simulink model "bit32cpu"  (R2020a)
settings: Solver=VariableStepAuto  StartTime=0.0  StopTime=10.0  RelTol=1e-3
libraries: simulink_extras x392
(part 10 of 63)

== system bit32cpu/ALU/Multiplier/Subsystem2/Subsystem1/Subsystem3 ==
  In1 : Inport
  In2 : Inport  Port=2
  In3 : Inport  Port=3
  In4 : Inport  Port=4
  In5 : Inport  Port=5
  In6 : Inport  Port=6
  In7 : Inport  Port=7
  In8 : Inport  Port=8
  Logical Operator{,1..15} (16 alike) : Logic  AllPortsSameDT=off  OutDataTypeStr=boolean
  Subsystem : Subsystem
  Subsystem1 : Subsystem
  Subsystem10 : Subsystem
  Subsystem11 : Subsystem
  Subsystem12 : Subsystem
  Subsystem13 : Subsystem
  Subsystem14 : Subsystem
  Subsystem2 : Subsystem
  Subsystem3 : Subsystem
  Subsystem4 : Subsystem
  Subsystem5 : Subsystem
  Subsystem6 : Subsystem
  Subsystem7 : Subsystem
  Subsystem8 : Subsystem
  Subsystem9 : Subsystem
  Out1 : Outport
  Out2 : Outport  Port=2
  Out3 : Outport  Port=3
  Out4 : Outport  Port=4
  Out5 : Outport  Port=5
  Out6 : Outport  Port=6
  Out7 : Outport  Port=7
  Out8 : Outport  Port=8
  Out9 : Outport  Port=9
  wires:
  Logical Operator3/1 -> Out9/1
  Subsystem2/1(Out1) -> Out7/1
  Logical Operator4/1 -> Subsystem6/1(In1)
  Subsystem1/2(Out2) -> Subsystem10/1(In1)
  Subsystem9/2(Out2) -> Subsystem14/2(In2)
  Subsystem7/1(Out1) -> Out5/1
  Logical Operator11/1 -> Subsystem1/3(In3)
  Logical Operator10/1 -> Subsystem3/3(In3)
  Subsystem4/1(Out1) -> Out6/1
  In4/1 -> Logical Operator15/2, Logical Operator11/2, Logical Operator7/2, Logical Operator3/2
  Subsystem14/1(Out1) -> Out2/1
  Subsystem14/2(Out2) -> Out1/1
  Logical Operator8/1 -> Subsystem8/1(In1)
  Subsystem3/2(Out2) -> Subsystem5/1(In1)
  In5/1 -> Logical Operator12/1, Logical Operator13/1, Logical Operator14/1, Logical Operator15/1
  In7/1 -> Logical Operator4/1, Logical Operator5/1, Logical Operator6/1, Logical Operator7/1
  Subsystem8/2(Out2) -> Subsystem12/1(In1)
  Subsystem13/1(Out1) -> Out4/1
  Subsystem/1(Out1) -> Out8/1
  Subsystem9/1(Out1) -> Out3/1
  Subsystem11/1(Out1) -> Subsystem8/3(In3)
  Logical Operator2/1 -> Subsystem/1(In1)
  In8/1 -> Logical Operator/1, Logical Operator1/1, Logical Operator2/1, Logical Operator3/1
  Logical Operator6/1 -> Subsystem1/2(In2)
  Subsystem12/1(Out1) -> Subsystem9/3(In3)
  In2/1 -> Logical Operator9/2, Logical Operator13/2, Logical Operator5/2, Logical Operator1/2
  Subsystem5/2(Out2) -> Subsystem13/2(In2)
  Logical Operator12/1 -> Subsystem9/1(In1)
  Subsystem2/2(Out2) -> Subsystem10/2(In2)
  Logical Operator14/1 -> Subsystem6/3(In3)
  In3/1 -> Logical Operator6/2, Logical Operator14/2, Logical Operator10/2, Logical Operator2/2
  Subsystem4/2(Out2) -> Subsystem5/2(In2)
  Subsystem/2(Out2) -> Subsystem2/2(In2)
  In1/1 -> Logical Operator12/2, Logical Operator8/2, Logical Operator4/2, Logical Operator/2
  In6/1 -> Logical Operator8/1, Logical Operator9/1, Logical Operator10/1, Logical Operator11/1
  Logical Operator/1 -> Subsystem3/1(In1)
  Logical Operator9/1 -> Subsystem6/2(In2)
  Subsystem12/2(Out2) -> Subsystem14/1(In1)
  Subsystem10/2(Out2) -> Subsystem7/3(In3)
  Logical Operator13/1 -> Subsystem8/2(In2)
  Logical Operator1/1 -> Subsystem1/1(In1)
  Subsystem1/1(Out1) -> Subsystem2/1(In1)
  Subsystem6/2(Out2) -> Subsystem11/1(In1)
  Logical Operator5/1 -> Subsystem3/2(In2)
  Logical Operator7/1 -> Subsystem/2(In2)
  Subsystem11/2(Out2) -> Subsystem9/2(In2)
  Subsystem6/1(Out1) -> Subsystem7/1(In1)
  Subsystem8/1(Out1) -> Subsystem13/1(In1)
  Subsystem13/2(Out2) -> Subsystem12/2(In2)
  Subsystem5/1(Out1) -> Subsystem7/2(In2)
  Logical Operator15/1 -> Subsystem4/1(In1)
  Subsystem3/1(Out1) -> Subsystem4/2(In2)
  Subsystem7/2(Out2) -> Subsystem11/2(In2)
  Subsystem10/1(Out1) -> Subsystem4/3(In3)

== system bit32cpu/ALU/Multiplier/Subsystem2/Subsystem1/Subsystem4 ==
  In1 : Inport
  In2 : Inport  Port=2
  In3 : Inport  Port=3
  In4 : Inport  Port=4
  In5 : Inport  Port=5
  In6 : Inport  Port=6
  In7 : Inport  Port=7
  In8 : Inport  Port=8
  In9 : Inport  Port=9
  In10 : Inport  Port=10
  In11 : Inport  Port=11
  In12 : Inport  Port=12
  In13 : Inport  Port=13
  In14 : Inport  Port=14
  In15 : Inport  Port=15
  In16 : Inport  Port=16
  Constant16 : Constant  Value=0
  Subsystem : Subsystem
  Subsystem4 : Subsystem
  Out1 : Outport
  Out2 : Outport  Port=2
  Out3 : Outport  Port=3
  Out4 : Outport  Port=4
  Out5 : Outport  Port=5
  Out6 : Outport  Port=6
  Out7 : Outport  Port=7
  Out8 : Outport  Port=8
  Out9 : Outport  Port=9
  wires:
  Subsystem/3(Out3) -> Out7/1
  Subsystem4/5(Out5) -> Out5/1
  Subsystem4/3(Out3) -> Out3/1
  Subsystem4/1(Out1) -> Out1/1
  Subsystem/2(Out2) -> Out6/1
  Subsystem4/2(Out2) -> Out2/1
  Subsystem/1(Out1) -> Subsystem4/5(In5)
  Subsystem4/4(Out4) -> Out4/1
  Subsystem/5(Out5) -> Out9/1
  Constant16/1 -> Subsystem/5(In5)
  Subsystem/4(Out4) -> Out8/1
  In1/1 -> Subsystem4/1(In1)
  In2/1 -> Subsystem4/2(In2)
  In3/1 -> Subsystem4/3(In3)
  In4/1 -> Subsystem4/4(In4)
  In5/1 -> Subsystem/1(In1)
  In6/1 -> Subsystem/2(In2)
  In7/1 -> Subsystem/3(In3)
  In8/1 -> Subsystem/4(In4)
  In9/1 -> Subsystem4/6(In6)
  In10/1 -> Subsystem4/7(In7)
  In11/1 -> Subsystem4/8(In8)
  In12/1 -> Subsystem4/9(In9)
  In13/1 -> Subsystem/6(In6)
  In14/1 -> Subsystem/7(In7)
  In15/1 -> Subsystem/8(In8)
  In16/1 -> Subsystem/9(In9)

== system bit32cpu/ALU/Multiplier/Subsystem2/Subsystem1/Subsystem5 ==
  In1 : Inport
  In2 : Inport  Port=2
  In3 : Inport  Port=3
  In4 : Inport  Port=4
  In5 : Inport  Port=5
  In6 : Inport  Port=6
  In7 : Inport  Port=7
  In8 : Inport  Port=8
  In9 : Inport  Port=9
  In10 : Inport  Port=10
  In11 : Inport  Port=11
  In12 : Inport  Port=12
  In13 : Inport  Port=13
  In14 : Inport  Port=14
  In15 : Inport  Port=15
  In16 : Inport  Port=16
  Constant16 : Constant  Value=0
  Subsystem : Subsystem
  Subsystem4 : Subsystem
  Out1 : Outport
  Out2 : Outport  Port=2
  Out3 : Outport  Port=3
  Out4 : Outport  Port=4
  Out5 : Outport  Port=5
  Out6 : Outport  Port=6
  Out7 : Outport  Port=7
  Out8 : Outport  Port=8
  Out9 : Outport  Port=9
  wires:
  Subsystem/3(Out3) -> Out7/1
  Subsystem4/5(Out5) -> Out5/1
  Subsystem4/3(Out3) -> Out3/1
  Subsystem4/1(Out1) -> Out1/1
  Subsystem/2(Out2) -> Out6/1
  Subsystem4/2(Out2) -> Out2/1
  Subsystem/1(Out1) -> Subsystem4/5(In5)
  Subsystem4/4(Out4) -> Out4/1
  Subsystem/5(Out5) -> Out9/1
  Constant16/1 -> Subsystem/5(In5)
  Subsystem/4(Out4) -> Out8/1
  In1/1 -> Subsystem4/1(In1)
  In2/1 -> Subsystem4/2(In2)
  In3/1 -> Subsystem4/3(In3)
  In4/1 -> Subsystem4/4(In4)
  In5/1 -> Subsystem/1(In1)
  In6/1 -> Subsystem/2(In2)
  In7/1 -> Subsystem/3(In3)
  In8/1 -> Subsystem/4(In4)
  In9/1 -> Subsystem4/6(In6)
  In10/1 -> Subsystem4/7(In7)
  In11/1 -> Subsystem4/8(In8)
  In12/1 -> Subsystem4/9(In9)
  In13/1 -> Subsystem/6(In6)
  In14/1 -> Subsystem/7(In7)
  In15/1 -> Subsystem/8(In8)
  In16/1 -> Subsystem/9(In9)

== system bit32cpu/ALU/Multiplier/Subsystem2/Subsystem1/Subsystem6 ==
  In1 : Inport
  In2 : Inport  Port=2
  In3 : Inport  Port=3
  In4 : Inport  Port=4
  In5 : Inport  Port=5
  In6 : Inport  Port=6
  In7 : Inport  Port=7
  In8 : Inport  Port=8
  In9 : Inport  Port=9
  In10 : Inport  Port=10
  In11 : Inport  Port=11
  In12 : Inport  Port=12
  In13 : Inport  Port=13
  In14 : Inport  Port=14
  In15 : Inport  Port=15
  In16 : Inport  Port=16
  Constant : Constant  Value=0
  Subsystem : Subsystem
  Subsystem4 : Subsystem
  Out1 : Outport
  Out2 : Outport  Port=2
  Out3 : Outport  Port=3
  Out4 : Outport  Port=4
  Out5 : Outport  Port=5
  Out6 : Outport  Port=6
  Out7 : Outport  Port=7
  Out8 : Outport  Port=8
  Out9 : Outport  Port=9
  wires:
  Subsystem/3(Out3) -> Out7/1
  Subsystem4/5(Out5) -> Out5/1
  Subsystem4/3(Out3) -> Out3/1
  Subsystem4/1(Out1) -> Out1/1
  Subsystem/2(Out2) -> Out6/1
  Subsystem4/2(Out2) -> Out2/1
  Subsystem/1(Out1) -> Subsystem4/5(In5)
  Subsystem4/4(Out4) -> Out4/1
  Subsystem/5(Out5) -> Out9/1
  Constant/1 -> Subsystem/5(In5)
  Subsystem/4(Out4) -> Out8/1
  In1/1 -> Subsystem4/1(In1)
  In2/1 -> Subsystem4/2(In2)
  In3/1 -> Subsystem4/3(In3)
  In4/1 -> Subsystem4/4(In4)
  In5/1 -> Subsystem/1(In1)
  In6/1 -> Subsystem/2(In2)
  In7/1 -> Subsystem/3(In3)
  In8/1 -> Subsystem/4(In4)
  In9/1 -> Subsystem4/6(In6)
  In10/1 -> Subsystem4/7(In7)
  In11/1 -> Subsystem4/8(In8)
  In12/1 -> Subsystem4/9(In9)
  In13/1 -> Subsystem/6(In6)
  In14/1 -> Subsystem/7(In7)
  In15/1 -> Subsystem/8(In8)
  In16/1 -> Subsystem/9(In9)

== system bit32cpu/ALU/Multiplier/Subsystem2/Subsystem2/Subsystem1 ==
  In1 : Inport
  In2 : Inport  Port=2
  In3 : Inport  Port=3
  In4 : Inport  Port=4
  In5 : Inport  Port=5
  In6 : Inport  Port=6
  In7 : Inport  Port=7
  In8 : Inport  Port=8
  Logical Operator{,1..15} (16 alike) : Logic  AllPortsSameDT=off  OutDataTypeStr=boolean
  Subsystem : Subsystem
  Subsystem1 : Subsystem
  Subsystem10 : Subsystem
  Subsystem11 : Subsystem
  Subsystem12 : Subsystem
  Subsystem13 : Subsystem
  Subsystem14 : Subsystem
  Subsystem2 : Subsystem
  Subsystem3 : Subsystem
  Subsystem4 : Subsystem
  Subsystem5 : Subsystem
  Subsystem6 : Subsystem
  Subsystem7 : Subsystem
  Subsystem8 : Subsystem
  Subsystem9 : Subsystem
  Out1 : Outport
  Out2 : Outport  Port=2
  Out3 : Outport  Port=3
  Out4 : Outport  Port=4
  Out5 : Outport  Port=5
  Out6 : Outport  Port=6
  Out7 : Outport  Port=7
  Out8 : Outport  Port=8
  Out9 : Outport  Port=9
  wires:
  Logical Operator3/1 -> Out9/1
  Subsystem2/1(Out1) -> Out7/1
  Logical Operator4/1 -> Subsystem6/1(In1)
  Subsystem1/2(Out2) -> Subsystem10/1(In1)
  Subsystem9/2(Out2) -> Subsystem14/2(In2)
  Subsystem7/1(Out1) -> Out5/1
  Logical Operator11/1 -> Subsystem1/3(In3)
  Logical Operator10/1 -> Subsystem3/3(In3)
  Subsystem4/1(Out1) -> Out6/1
  In4/1 -> Logical Operator15/2, Logical Operator11/2, Logical Operator7/2, Logical Operator3/2
  Subsystem14/1(Out1) -> Out2/1
  Subsystem14/2(Out2) -> Out1/1
  Logical Operator8/1 -> Subsystem8/1(In1)
  Subsystem3/2(Out2) -> Subsystem5/1(In1)
  In5/1 -> Logical Operator12/1, Logical Operator13/1, Logical Operator14/1, Logical Operator15/1
  In7/1 -> Logical Operator4/1, Logical Operator5/1, Logical Operator6/1, Logical Operator7/1
  Subsystem8/2(Out2) -> Subsystem12/1(In1)
  Subsystem13/1(Out1) -> Out4/1
  Subsystem/1(Out1) -> Out8/1
  Subsystem9/1(Out1) -> Out3/1
  Subsystem11/1(Out1) -> Subsystem8/3(In3)
  Logical Operator2/1 -> Subsystem/1(In1)
  In8/1 -> Logical Operator/1, Logical Operator1/1, Logical Operator2/1, Logical Operator3/1
  Logical Operator6/1 -> Subsystem1/2(In2)
  Subsystem12/1(Out1) -> Subsystem9/3(In3)
  In2/1 -> Logical Operator9/2, Logical Operator13/2, Logical Operator5/2, Logical Operator1/2
  Subsystem5/2(Out2) -> Subsystem13/2(In2)
  Logical Operator12/1 -> Subsystem9/1(In1)
  Subsystem2/2(Out2) -> Subsystem10/2(In2)
  Logical Operator14/1 -> Subsystem6/3(In3)
  In3/1 -> Logical Operator6/2, Logical Operator14/2, Logical Operator10/2, Logical Operator2/2
  Subsystem4/2(Out2) -> Subsystem5/2(In2)
  Subsystem/2(Out2) -> Subsystem2/2(In2)
  In1/1 -> Logical Operator12/2, Logical Operator8/2, Logical Operator4/2, Logical Operator/2
  In6/1 -> Logical Operator8/1, Logical Operator9/1, Logical Operator10/1, Logical Operator11/1
  Logical Operator/1 -> Subsystem3/1(In1)
  Logical Operator9/1 -> Subsystem6/2(In2)
  Subsystem12/2(Out2) -> Subsystem14/1(In1)
  Subsystem10/2(Out2) -> Subsystem7/3(In3)
  Logical Operator13/1 -> Subsystem8/2(In2)
  Logical Operator1/1 -> Subsystem1/1(In1)
  Subsystem1/1(Out1) -> Subsystem2/1(In1)
  Subsystem6/2(Out2) -> Subsystem11/1(In1)
  Logical Operator5/1 -> Subsystem3/2(In2)
  Logical Operator7/1 -> Subsystem/2(In2)
  Subsystem11/2(Out2) -> Subsystem9/2(In2)
  Subsystem6/1(Out1) -> Subsystem7/1(In1)
  Subsystem8/1(Out1) -> Subsystem13/1(In1)
  Subsystem13/2(Out2) -> Subsystem12/2(In2)
  Subsystem5/1(Out1) -> Subsystem7/2(In2)
  Logical Operator15/1 -> Subsystem4/1(In1)
  Subsystem3/1(Out1) -> Subsystem4/2(In2)
  Subsystem7/2(Out2) -> Subsystem11/2(In2)
  Subsystem10/1(Out1) -> Subsystem4/3(In3)

== system bit32cpu/ALU/Multiplier/Subsystem2/Subsystem2/Subsystem15 ==
  In1 : Inport
  In2 : Inport  Port=2
  In3 : Inport  Port=3
  In4 : Inport  Port=4
  In5 : Inport  Port=5
  In6 : Inport  Port=6
  In7 : Inport  Port=7
  In8 : Inport  Port=8
  Logical Operator{,1..15} (16 alike) : Logic  AllPortsSameDT=off  OutDataTypeStr=boolean
  Subsystem : Subsystem
  Subsystem1 : Subsystem
  Subsystem10 : Subsystem
  Subsystem11 : Subsystem
  Subsystem12 : Subsystem
  Subsystem13 : Subsystem
  Subsystem14 : Subsystem
  Subsystem2 : Subsystem
  Subsystem3 : Subsystem
  Subsystem4 : Subsystem
  Subsystem5 : Subsystem
  Subsystem6 : Subsystem
  Subsystem7 : Subsystem
  Subsystem8 : Subsystem
  Subsystem9 : Subsystem
  Out1 : Outport
  Out2 : Outport  Port=2
  Out3 : Outport  Port=3
  Out4 : Outport  Port=4
  Out5 : Outport  Port=5
  Out6 : Outport  Port=6
  Out7 : Outport  Port=7
  Out8 : Outport  Port=8
  Out9 : Outport  Port=9
  wires:
  Logical Operator3/1 -> Out9/1
  Subsystem2/1(Out1) -> Out7/1
  Logical Operator4/1 -> Subsystem6/1(In1)
  Subsystem1/2(Out2) -> Subsystem10/1(In1)
  Subsystem9/2(Out2) -> Subsystem14/2(In2)
  Subsystem7/1(Out1) -> Out5/1
  Logical Operator11/1 -> Subsystem1/3(In3)
  Logical Operator10/1 -> Subsystem3/3(In3)
  Subsystem4/1(Out1) -> Out6/1
  In4/1 -> Logical Operator15/2, Logical Operator11/2, Logical Operator7/2, Logical Operator3/2
  Subsystem14/1(Out1) -> Out2/1
  Subsystem14/2(Out2) -> Out1/1
  Logical Operator8/1 -> Subsystem8/1(In1)
  Subsystem3/2(Out2) -> Subsystem5/1(In1)
  In5/1 -> Logical Operator12/1, Logical Operator13/1, Logical Operator14/1, Logical Operator15/1
  In7/1 -> Logical Operator4/1, Logical Operator5/1, Logical Operator6/1, Logical Operator7/1
  Subsystem8/2(Out2) -> Subsystem12/1(In1)
  Subsystem13/1(Out1) -> Out4/1
  Subsystem/1(Out1) -> Out8/1
  Subsystem9/1(Out1) -> Out3/1
  Subsystem11/1(Out1) -> Subsystem8/3(In3)
  Logical Operator2/1 -> Subsystem/1(In1)
  In8/1 -> Logical Operator/1, Logical Operator1/1, Logical Operator2/1, Logical Operator3/1
  Logical Operator6/1 -> Subsystem1/2(In2)
  Subsystem12/1(Out1) -> Subsystem9/3(In3)
  In2/1 -> Logical Operator9/2, Logical Operator13/2, Logical Operator5/2, Logical Operator1/2
  Subsystem5/2(Out2) -> Subsystem13/2(In2)
  Logical Operator12/1 -> Subsystem9/1(In1)
  Subsystem2/2(Out2) -> Subsystem10/2(In2)
  Logical Operator14/1 -> Subsystem6/3(In3)
  In3/1 -> Logical Operator6/2, Logical Operator14/2, Logical Operator10/2, Logical Operator2/2
  Subsystem4/2(Out2) -> Subsystem5/2(In2)
  Subsystem/2(Out2) -> Subsystem2/2(In2)
  In1/1 -> Logical Operator12/2, Logical Operator8/2, Logical Operator4/2, Logical Operator/2
  In6/1 -> Logical Operator8/1, Logical Operator9/1, Logical Operator10/1, Logical Operator11/1
  Logical Operator/1 -> Subsystem3/1(In1)
  Logical Operator9/1 -> Subsystem6/2(In2)
  Subsystem12/2(Out2) -> Subsystem14/1(In1)
  Subsystem10/2(Out2) -> Subsystem7/3(In3)
  Logical Operator13/1 -> Subsystem8/2(In2)
  Logical Operator1/1 -> Subsystem1/1(In1)
  Subsystem1/1(Out1) -> Subsystem2/1(In1)
  Subsystem6/2(Out2) -> Subsystem11/1(In1)
  Logical Operator5/1 -> Subsystem3/2(In2)
  Logical Operator7/1 -> Subsystem/2(In2)
  Subsystem11/2(Out2) -> Subsystem9/2(In2)
  Subsystem6/1(Out1) -> Subsystem7/1(In1)
  Subsystem8/1(Out1) -> Subsystem13/1(In1)
  Subsystem13/2(Out2) -> Subsystem12/2(In2)
  Subsystem5/1(Out1) -> Subsystem7/2(In2)
  Logical Operator15/1 -> Subsystem4/1(In1)
  Subsystem3/1(Out1) -> Subsystem4/2(In2)
  Subsystem7/2(Out2) -> Subsystem11/2(In2)
  Subsystem10/1(Out1) -> Subsystem4/3(In3)

== system bit32cpu/ALU/Multiplier/Subsystem2/Subsystem2/Subsystem2 ==
  In1 : Inport
  In2 : Inport  Port=2
  In3 : Inport  Port=3
  In4 : Inport  Port=4
  In5 : Inport  Port=5
  In6 : Inport  Port=6
  In7 : Inport  Port=7
  In8 : Inport  Port=8
  Logical Operator{,1..15} (16 alike) : Logic  AllPortsSameDT=off  OutDataTypeStr=boolean
  Subsystem : Subsystem
  Subsystem1 : Subsystem
  Subsystem10 : Subsystem
  Subsystem11 : Subsystem
  Subsystem12 : Subsystem
  Subsystem13 : Subsystem
  Subsystem14 : Subsystem
  Subsystem2 : Subsystem
  Subsystem3 : Subsystem
  Subsystem4 : Subsystem
  Subsystem5 : Subsystem
  Subsystem6 : Subsystem
  Subsystem7 : Subsystem
  Subsystem8 : Subsystem
  Subsystem9 : Subsystem
  Out1 : Outport
  Out2 : Outport  Port=2
  Out3 : Outport  Port=3
  Out4 : Outport  Port=4
  Out5 : Outport  Port=5
  Out6 : Outport  Port=6
  Out7 : Outport  Port=7
  Out8 : Outport  Port=8
  Out9 : Outport  Port=9
  wires:
  Logical Operator3/1 -> Out9/1
  Subsystem2/1(Out1) -> Out7/1
  Logical Operator4/1 -> Subsystem6/1(In1)
  Subsystem1/2(Out2) -> Subsystem10/1(In1)
  Subsystem9/2(Out2) -> Subsystem14/2(In2)
  Subsystem7/1(Out1) -> Out5/1
  Logical Operator11/1 -> Subsystem1/3(In3)
  Logical Operator10/1 -> Subsystem3/3(In3)
  Subsystem4/1(Out1) -> Out6/1
  In4/1 -> Logical Operator15/2, Logical Operator11/2, Logical Operator7/2, Logical Operator3/2
  Subsystem14/1(Out1) -> Out2/1
  Subsystem14/2(Out2) -> Out1/1
  Logical Operator8/1 -> Subsystem8/1(In1)
  Subsystem3/2(Out2) -> Subsystem5/1(In1)
  In5/1 -> Logical Operator12/1, Logical Operator13/1, Logical Operator14/1, Logical Operator15/1
  In7/1 -> Logical Operator4/1, Logical Operator5/1, Logical Operator6/1, Logical Operator7/1
  Subsystem8/2(Out2) -> Subsystem12/1(In1)
  Subsystem13/1(Out1) -> Out4/1
  Subsystem/1(Out1) -> Out8/1
  Subsystem9/1(Out1) -> Out3/1
  Subsystem11/1(Out1) -> Subsystem8/3(In3)
  Logical Operator2/1 -> Subsystem/1(In1)
  In8/1 -> Logical Operator/1, Logical Operator1/1, Logical Operator2/1, Logical Operator3/1
  Logical Operator6/1 -> Subsystem1/2(In2)
  Subsystem12/1(Out1) -> Subsystem9/3(In3)
  In2/1 -> Logical Operator9/2, Logical Operator13/2, Logical Operator5/2, Logical Operator1/2
  Subsystem5/2(Out2) -> Subsystem13/2(In2)
  Logical Operator12/1 -> Subsystem9/1(In1)
  Subsystem2/2(Out2) -> Subsystem10/2(In2)
  Logical Operator14/1 -> Subsystem6/3(In3)
  In3/1 -> Logical Operator6/2, Logical Operator14/2, Logical Operator10/2, Logical Operator2/2
  Subsystem4/2(Out2) -> Subsystem5/2(In2)
  Subsystem/2(Out2) -> Subsystem2/2(In2)
  In1/1 -> Logical Operator12/2, Logical Operator8/2, Logical Operator4/2, Logical Operator/2
  In6/1 -> Logical Operator8/1, Logical Operator9/1, Logical Operator10/1, Logical Operator11/1
  Logical Operator/1 -> Subsystem3/1(In1)
  Logical Operator9/1 -> Subsystem6/2(In2)
  Subsystem12/2(Out2) -> Subsystem14/1(In1)
  Subsystem10/2(Out2) -> Subsystem7/3(In3)
  Logical Operator13/1 -> Subsystem8/2(In2)
  Logical Operator1/1 -> Subsystem1/1(In1)
  Subsystem1/1(Out1) -> Subsystem2/1(In1)
  Subsystem6/2(Out2) -> Subsystem11/1(In1)
  Logical Operator5/1 -> Subsystem3/2(In2)
  Logical Operator7/1 -> Subsystem/2(In2)
  Subsystem11/2(Out2) -> Subsystem9/2(In2)
  Subsystem6/1(Out1) -> Subsystem7/1(In1)
  Subsystem8/1(Out1) -> Subsystem13/1(In1)
  Subsystem13/2(Out2) -> Subsystem12/2(In2)
  Subsystem5/1(Out1) -> Subsystem7/2(In2)
  Logical Operator15/1 -> Subsystem4/1(In1)
  Subsystem3/1(Out1) -> Subsystem4/2(In2)
  Subsystem7/2(Out2) -> Subsystem11/2(In2)
  Subsystem10/1(Out1) -> Subsystem4/3(In3)

== system bit32cpu/ALU/Multiplier/Subsystem2/Subsystem2/Subsystem3 ==
  In1 : Inport
  In2 : Inport  Port=2
  In3 : Inport  Port=3
  In4 : Inport  Port=4
  In5 : Inport  Port=5
  In6 : Inport  Port=6
  In7 : Inport  Port=7
  In8 : Inport  Port=8
  Logical Operator{,1..15} (16 alike) : Logic  AllPortsSameDT=off  OutDataTypeStr=boolean
  Subsystem : Subsystem
  Subsystem1 : Subsystem
  Subsystem10 : Subsystem
  Subsystem11 : Subsystem
  Subsystem12 : Subsystem
  Subsystem13 : Subsystem
  Subsystem14 : Subsystem
  Subsystem2 : Subsystem
  Subsystem3 : Subsystem
  Subsystem4 : Subsystem
  Subsystem5 : Subsystem
  Subsystem6 : Subsystem
  Subsystem7 : Subsystem
  Subsystem8 : Subsystem
  Subsystem9 : Subsystem
  Out1 : Outport
  Out2 : Outport  Port=2
  Out3 : Outport  Port=3
  Out4 : Outport  Port=4
  Out5 : Outport  Port=5
  Out6 : Outport  Port=6
  Out7 : Outport  Port=7
  Out8 : Outport  Port=8
  Out9 : Outport  Port=9
  wires:
  Logical Operator3/1 -> Out9/1
  Subsystem2/1(Out1) -> Out7/1
  Logical Operator4/1 -> Subsystem6/1(In1)
  Subsystem1/2(Out2) -> Subsystem10/1(In1)
  Subsystem9/2(Out2) -> Subsystem14/2(In2)
  Subsystem7/1(Out1) -> Out5/1
  Logical Operator11/1 -> Subsystem1/3(In3)
  Logical Operator10/1 -> Subsystem3/3(In3)
  Subsystem4/1(Out1) -> Out6/1
  In4/1 -> Logical Operator15/2, Logical Operator11/2, Logical Operator7/2, Logical Operator3/2
  Subsystem14/1(Out1) -> Out2/1
  Subsystem14/2(Out2) -> Out1/1
  Logical Operator8/1 -> Subsystem8/1(In1)
  Subsystem3/2(Out2) -> Subsystem5/1(In1)
  In5/1 -> Logical Operator12/1, Logical Operator13/1, Logical Operator14/1, Logical Operator15/1
  In7/1 -> Logical Operator4/1, Logical Operator5/1, Logical Operator6/1, Logical Operator7/1
  Subsystem8/2(Out2) -> Subsystem12/1(In1)
  Subsystem13/1(Out1) -> Out4/1
  Subsystem/1(Out1) -> Out8/1
  Subsystem9/1(Out1) -> Out3/1
  Subsystem11/1(Out1) -> Subsystem8/3(In3)
  Logical Operator2/1 -> Subsystem/1(In1)
  In8/1 -> Logical Operator/1, Logical Operator1/1, Logical Operator2/1, Logical Operator3/1
  Logical Operator6/1 -> Subsystem1/2(In2)
  Subsystem12/1(Out1) -> Subsystem9/3(In3)
  In2/1 -> Logical Operator9/2, Logical Operator13/2, Logical Operator5/2, Logical Operator1/2
  Subsystem5/2(Out2) -> Subsystem13/2(In2)
  Logical Operator12/1 -> Subsystem9/1(In1)
  Subsystem2/2(Out2) -> Subsystem10/2(In2)
  Logical Operator14/1 -> Subsystem6/3(In3)
  In3/1 -> Logical Operator6/2, Logical Operator14/2, Logical Operator10/2, Logical Operator2/2
  Subsystem4/2(Out2) -> Subsystem5/2(In2)
  Subsystem/2(Out2) -> Subsystem2/2(In2)
  In1/1 -> Logical Operator12/2, Logical Operator8/2, Logical Operator4/2, Logical Operator/2
  In6/1 -> Logical Operator8/1, Logical Operator9/1, Logical Operator10/1, Logical Operator11/1
  Logical Operator/1 -> Subsystem3/1(In1)
  Logical Operator9/1 -> Subsystem6/2(In2)
  Subsystem12/2(Out2) -> Subsystem14/1(In1)
  Subsystem10/2(Out2) -> Subsystem7/3(In3)
  Logical Operator13/1 -> Subsystem8/2(In2)
  Logical Operator1/1 -> Subsystem1/1(In1)
  Subsystem1/1(Out1) -> Subsystem2/1(In1)
  Subsystem6/2(Out2) -> Subsystem11/1(In1)
  Logical Operator5/1 -> Subsystem3/2(In2)
  Logical Operator7/1 -> Subsystem/2(In2)
  Subsystem11/2(Out2) -> Subsystem9/2(In2)
  Subsystem6/1(Out1) -> Subsystem7/1(In1)
  Subsystem8/1(Out1) -> Subsystem13/1(In1)
  Subsystem13/2(Out2) -> Subsystem12/2(In2)
  Subsystem5/1(Out1) -> Subsystem7/2(In2)
  Logical Operator15/1 -> Subsystem4/1(In1)
  Subsystem3/1(Out1) -> Subsystem4/2(In2)
  Subsystem7/2(Out2) -> Subsystem11/2(In2)
  Subsystem10/1(Out1) -> Subsystem4/3(In3)

== system bit32cpu/ALU/Multiplier/Subsystem2/Subsystem2/Subsystem4 ==
  In1 : Inport
  In2 : Inport  Port=2
  In3 : Inport  Port=3
  In4 : Inport  Port=4
  In5 : Inport  Port=5
  In6 : Inport  Port=6
  In7 : Inport  Port=7
  In8 : Inport  Port=8
  In9 : Inport  Port=9
  In10 : Inport  Port=10
  In11 : Inport  Port=11
  In12 : Inport  Port=12
  In13 : Inport  Port=13
  In14 : Inport  Port=14
  In15 : Inport  Port=15
  In16 : Inport  Port=16
  Constant16 : Constant  Value=0
  Subsystem : Subsystem
  Subsystem4 : Subsystem
  Out1 : Outport
  Out2 : Outport  Port=2
  Out3 : Outport  Port=3
  Out4 : Outport  Port=4
  Out5 : Outport  Port=5
  Out6 : Outport  Port=6
  Out7 : Outport  Port=7
  Out8 : Outport  Port=8
  Out9 : Outport  Port=9
  wires:
  Subsystem/3(Out3) -> Out7/1
  Subsystem4/5(Out5) -> Out5/1
  Subsystem4/3(Out3) -> Out3/1
  Subsystem4/1(Out1) -> Out1/1
  Subsystem/2(Out2) -> Out6/1
  Subsystem4/2(Out2) -> Out2/1
  Subsystem/1(Out1) -> Subsystem4/5(In5)
  Subsystem4/4(Out4) -> Out4/1
  Subsystem/5(Out5) -> Out9/1
  Constant16/1 -> Subsystem/5(In5)
  Subsystem/4(Out4) -> Out8/1
  In1/1 -> Subsystem4/1(In1)
  In2/1 -> Subsystem4/2(In2)
  In3/1 -> Subsystem4/3(In3)
  In4/1 -> Subsystem4/4(In4)
  In5/1 -> Subsystem/1(In1)
  In6/1 -> Subsystem/2(In2)
  In7/1 -> Subsystem/3(In3)
  In8/1 -> Subsystem/4(In4)
  In9/1 -> Subsystem4/6(In6)
  In10/1 -> Subsystem4/7(In7)
  In11/1 -> Subsystem4/8(In8)
  In12/1 -> Subsystem4/9(In9)
  In13/1 -> Subsystem/6(In6)
  In14/1 -> Subsystem/7(In7)
  In15/1 -> Subsystem/8(In8)
  In16/1 -> Subsystem/9(In9)

== system bit32cpu/ALU/Multiplier/Subsystem2/Subsystem2/Subsystem5 ==
  In1 : Inport
  In2 : Inport  Port=2
  In3 : Inport  Port=3
  In4 : Inport  Port=4
  In5 : Inport  Port=5
  In6 : Inport  Port=6
  In7 : Inport  Port=7
  In8 : Inport  Port=8
  In9 : Inport  Port=9
  In10 : Inport  Port=10
  In11 : Inport  Port=11
  In12 : Inport  Port=12
  In13 : Inport  Port=13
  In14 : Inport  Port=14
  In15 : Inport  Port=15
  In16 : Inport  Port=16
  Constant16 : Constant  Value=0
  Subsystem : Subsystem
  Subsystem4 : Subsystem
  Out1 : Outport
  Out2 : Outport  Port=2
  Out3 : Outport  Port=3
  Out4 : Outport  Port=4
  Out5 : Outport  Port=5
  Out6 : Outport  Port=6
  Out7 : Outport  Port=7
  Out8 : Outport  Port=8
  Out9 : Outport  Port=9
  wires:
  Subsystem/3(Out3) -> Out7/1
  Subsystem4/5(Out5) -> Out5/1
  Subsystem4/3(Out3) -> Out3/1
  Subsystem4/1(Out1) -> Out1/1
  Subsystem/2(Out2) -> Out6/1
  Subsystem4/2(Out2) -> Out2/1
  Subsystem/1(Out1) -> Subsystem4/5(In5)
  Subsystem4/4(Out4) -> Out4/1
  Subsystem/5(Out5) -> Out9/1
  Constant16/1 -> Subsystem/5(In5)
  Subsystem/4(Out4) -> Out8/1
  In1/1 -> Subsystem4/1(In1)
  In2/1 -> Subsystem4/2(In2)
  In3/1 -> Subsystem4/3(In3)
  In4/1 -> Subsystem4/4(In4)
  In5/1 -> Subsystem/1(In1)
  In6/1 -> Subsystem/2(In2)
  In7/1 -> Subsystem/3(In3)
  In8/1 -> Subsystem/4(In4)
  In9/1 -> Subsystem4/6(In6)
  In10/1 -> Subsystem4/7(In7)
  In11/1 -> Subsystem4/8(In8)
  In12/1 -> Subsystem4/9(In9)
  In13/1 -> Subsystem/6(In6)
  In14/1 -> Subsystem/7(In7)
  In15/1 -> Subsystem/8(In8)
  In16/1 -> Subsystem/9(In9)

== system bit32cpu/ALU/Multiplier/Subsystem2/Subsystem2/Subsystem6 ==
  In1 : Inport
  In2 : Inport  Port=2
  In3 : Inport  Port=3
  In4 : Inport  Port=4
  In5 : Inport  Port=5
  In6 : Inport  Port=6
  In7 : Inport  Port=7
  In8 : Inport  Port=8
  In9 : Inport  Port=9
  In10 : Inport  Port=10
  In11 : Inport  Port=11
  In12 : Inport  Port=12
  In13 : Inport  Port=13
  In14 : Inport  Port=14
  In15 : Inport  Port=15
  In16 : Inport  Port=16
  Constant : Constant  Value=0
  Subsystem : Subsystem
  Subsystem4 : Subsystem
  Out1 : Outport
  Out2 : Outport  Port=2
  Out3 : Outport  Port=3
  Out4 : Outport  Port=4
  Out5 : Outport  Port=5
  Out6 : Outport  Port=6
  Out7 : Outport  Port=7
  Out8 : Outport  Port=8
  Out9 : Outport  Port=9
  wires:
  Subsystem/3(Out3) -> Out7/1
  Subsystem4/5(Out5) -> Out5/1
  Subsystem4/3(Out3) -> Out3/1
  Subsystem4/1(Out1) -> Out1/1
  Subsystem/2(Out2) -> Out6/1
  Subsystem4/2(Out2) -> Out2/1
  Subsystem/1(Out1) -> Subsystem4/5(In5)
  Subsystem4/4(Out4) -> Out4/1
  Subsystem/5(Out5) -> Out9/1
  Constant/1 -> Subsystem/5(In5)
  Subsystem/4(Out4) -> Out8/1
  In1/1 -> Subsystem4/1(In1)
  In2/1 -> Subsystem4/2(In2)
  In3/1 -> Subsystem4/3(In3)
  In4/1 -> Subsystem4/4(In4)
  In5/1 -> Subsystem/1(In1)
  In6/1 -> Subsystem/2(In2)
  In7/1 -> Subsystem/3(In3)
  In8/1 -> Subsystem/4(In4)
  In9/1 -> Subsystem4/6(In6)
  In10/1 -> Subsystem4/7(In7)
  In11/1 -> Subsystem4/8(In8)
  In12/1 -> Subsystem4/9(In9)
  In13/1 -> Subsystem/6(In6)
  In14/1 -> Subsystem/7(In7)
  In15/1 -> Subsystem/8(In8)
  In16/1 -> Subsystem/9(In9)

== system bit32cpu/ALU/Multiplier/Subsystem2/Subsystem3/Subsystem1 ==
  In1 : Inport
  In2 : Inport  Port=2
  In3 : Inport  Port=3
  In4 : Inport  Port=4
  In5 : Inport  Port=5
  In6 : Inport  Port=6
  In7 : Inport  Port=7
  In8 : Inport  Port=8
  Logical Operator{,1..15} (16 alike) : Logic  AllPortsSameDT=off  OutDataTypeStr=boolean
  Subsystem : Subsystem
  Subsystem1 : Subsystem
  Subsystem10 : Subsystem
  Subsystem11 : Subsystem
  Subsystem12 : Subsystem
  Subsystem13 : Subsystem
  Subsystem14 : Subsystem
  Subsystem2 : Subsystem
  Subsystem3 : Subsystem
  Subsystem4 : Subsystem
  Subsystem5 : Subsystem
  Subsystem6 : Subsystem
  Subsystem7 : Subsystem
  Subsystem8 : Subsystem
  Subsystem9 : Subsystem
  Out1 : Outport
  Out2 : Outport  Port=2
  Out3 : Outport  Port=3
  Out4 : Outport  Port=4
  Out5 : Outport  Port=5
  Out6 : Outport  Port=6
  Out7 : Outport  Port=7
  Out8 : Outport  Port=8
  Out9 : Outport  Port=9
  wires:
  Logical Operator3/1 -> Out9/1
  Subsystem2/1(Out1) -> Out7/1
  Logical Operator4/1 -> Subsystem6/1(In1)
  Subsystem1/2(Out2) -> Subsystem10/1(In1)
  Subsystem9/2(Out2) -> Subsystem14/2(In2)
  Subsystem7/1(Out1) -> Out5/1
  Logical Operator11/1 -> Subsystem1/3(In3)
  Logical Operator10/1 -> Subsystem3/3(In3)
  Subsystem4/1(Out1) -> Out6/1
  In4/1 -> Logical Operator15/2, Logical Operator11/2, Logical Operator7/2, Logical Operator3/2
  Subsystem14/1(Out1) -> Out2/1
  Subsystem14/2(Out2) -> Out1/1
  Logical Operator8/1 -> Subsystem8/1(In1)
  Subsystem3/2(Out2) -> Subsystem5/1(In1)
  In5/1 -> Logical Operator12/1, Logical Operator13/1, Logical Operator14/1, Logical Operator15/1
  In7/1 -> Logical Operator4/1, Logical Operator5/1, Logical Operator6/1, Logical Operator7/1
  Subsystem8/2(Out2) -> Subsystem12/1(In1)
  Subsystem13/1(Out1) -> Out4/1
  Subsystem/1(Out1) -> Out8/1
  Subsystem9/1(Out1) -> Out3/1
  Subsystem11/1(Out1) -> Subsystem8/3(In3)
  Logical Operator2/1 -> Subsystem/1(In1)
  In8/1 -> Logical Operator/1, Logical Operator1/1, Logical Operator2/1, Logical Operator3/1
  Logical Operator6/1 -> Subsystem1/2(In2)
  Subsystem12/1(Out1) -> Subsystem9/3(In3)
  In2/1 -> Logical Operator9/2, Logical Operator13/2, Logical Operator5/2, Logical Operator1/2
  Subsystem5/2(Out2) -> Subsystem13/2(In2)
  Logical Operator12/1 -> Subsystem9/1(In1)
  Subsystem2/2(Out2) -> Subsystem10/2(In2)
  Logical Operator14/1 -> Subsystem6/3(In3)
  In3/1 -> Logical Operator6/2, Logical Operator14/2, Logical Operator10/2, Logical Operator2/2
  Subsystem4/2(Out2) -> Subsystem5/2(In2)
  Subsystem/2(Out2) -> Subsystem2/2(In2)
  In1/1 -> Logical Operator12/2, Logical Operator8/2, Logical Operator4/2, Logical Operator/2
  In6/1 -> Logical Operator8/1, Logical Operator9/1, Logical Operator10/1, Logical Operator11/1
  Logical Operator/1 -> Subsystem3/1(In1)
  Logical Operator9/1 -> Subsystem6/2(In2)
  Subsystem12/2(Out2) -> Subsystem14/1(In1)
  Subsystem10/2(Out2) -> Subsystem7/3(In3)
  Logical Operator13/1 -> Subsystem8/2(In2)
  Logical Operator1/1 -> Subsystem1/1(In1)
  Subsystem1/1(Out1) -> Subsystem2/1(In1)
  Subsystem6/2(Out2) -> Subsystem11/1(In1)
  Logical Operator5/1 -> Subsystem3/2(In2)
  Logical Operator7/1 -> Subsystem/2(In2)
  Subsystem11/2(Out2) -> Subsystem9/2(In2)
  Subsystem6/1(Out1) -> Subsystem7/1(In1)
  Subsystem8/1(Out1) -> Subsystem13/1(In1)
  Subsystem13/2(Out2) -> Subsystem12/2(In2)
  Subsystem5/1(Out1) -> Subsystem7/2(In2)
  Logical Operator15/1 -> Subsystem4/1(In1)
  Subsystem3/1(Out1) -> Subsystem4/2(In2)
  Subsystem7/2(Out2) -> Subsystem11/2(In2)
  Subsystem10/1(Out1) -> Subsystem4/3(In3)

== system bit32cpu/ALU/Multiplier/Subsystem2/Subsystem3/Subsystem15 ==
  In1 : Inport
  In2 : Inport  Port=2
  In3 : Inport  Port=3
  In4 : Inport  Port=4
  In5 : Inport  Port=5
  In6 : Inport  Port=6
  In7 : Inport  Port=7
  In8 : Inport  Port=8
  Logical Operator{,1..15} (16 alike) : Logic  AllPortsSameDT=off  OutDataTypeStr=boolean
  Subsystem : Subsystem
  Subsystem1 : Subsystem
  Subsystem10 : Subsystem
  Subsystem11 : Subsystem
  Subsystem12 : Subsystem
  Subsystem13 : Subsystem
  Subsystem14 : Subsystem
  Subsystem2 : Subsystem
  Subsystem3 : Subsystem
  Subsystem4 : Subsystem
  Subsystem5 : Subsystem
  Subsystem6 : Subsystem
  Subsystem7 : Subsystem
  Subsystem8 : Subsystem
  Subsystem9 : Subsystem
  Out1 : Outport
  Out2 : Outport  Port=2
  Out3 : Outport  Port=3
  Out4 : Outport  Port=4
  Out5 : Outport  Port=5
  Out6 : Outport  Port=6
  Out7 : Outport  Port=7
  Out8 : Outport  Port=8
  Out9 : Outport  Port=9
  wires:
  Logical Operator3/1 -> Out9/1
  Subsystem2/1(Out1) -> Out7/1
  Logical Operator4/1 -> Subsystem6/1(In1)
  Subsystem1/2(Out2) -> Subsystem10/1(In1)
  Subsystem9/2(Out2) -> Subsystem14/2(In2)
  Subsystem7/1(Out1) -> Out5/1
  Logical Operator11/1 -> Subsystem1/3(In3)
  Logical Operator10/1 -> Subsystem3/3(In3)
  Subsystem4/1(Out1) -> Out6/1
  In4/1 -> Logical Operator15/2, Logical Operator11/2, Logical Operator7/2, Logical Operator3/2
  Subsystem14/1(Out1) -> Out2/1
  Subsystem14/2(Out2) -> Out1/1
  Logical Operator8/1 -> Subsystem8/1(In1)
  Subsystem3/2(Out2) -> Subsystem5/1(In1)
  In5/1 -> Logical Operator12/1, Logical Operator13/1, Logical Operator14/1, Logical Operator15/1
  In7/1 -> Logical Operator4/1, Logical Operator5/1, Logical Operator6/1, Logical Operator7/1
  Subsystem8/2(Out2) -> Subsystem12/1(In1)
  Subsystem13/1(Out1) -> Out4/1
  Subsystem/1(Out1) -> Out8/1
  Subsystem9/1(Out1) -> Out3/1
  Subsystem11/1(Out1) -> Subsystem8/3(In3)
  Logical Operator2/1 -> Subsystem/1(In1)
  In8/1 -> Logical Operator/1, Logical Operator1/1, Logical Operator2/1, Logical Operator3/1
  Logical Operator6/1 -> Subsystem1/2(In2)
  Subsystem12/1(Out1) -> Subsystem9/3(In3)
  In2/1 -> Logical Operator9/2, Logical Operator13/2, Logical Operator5/2, Logical Operator1/2
  Subsystem5/2(Out2) -> Subsystem13/2(In2)
  Logical Operator12/1 -> Subsystem9/1(In1)
  Subsystem2/2(Out2) -> Subsystem10/2(In2)
  Logical Operator14/1 -> Subsystem6/3(In3)
  In3/1 -> Logical Operator6/2, Logical Operator14/2, Logical Operator10/2, Logical Operator2/2
  Subsystem4/2(Out2) -> Subsystem5/2(In2)
  Subsystem/2(Out2) -> Subsystem2/2(In2)
  In1/1 -> Logical Operator12/2, Logical Operator8/2, Logical Operator4/2, Logical Operator/2
  In6/1 -> Logical Operator8/1, Logical Operator9/1, Logical Operator10/1, Logical Operator11/1
  Logical Operator/1 -> Subsystem3/1(In1)
  Logical Operator9/1 -> Subsystem6/2(In2)
  Subsystem12/2(Out2) -> Subsystem14/1(In1)
  Subsystem10/2(Out2) -> Subsystem7/3(In3)
  Logical Operator13/1 -> Subsystem8/2(In2)
  Logical Operator1/1 -> Subsystem1/1(In1)
  Subsystem1/1(Out1) -> Subsystem2/1(In1)
  Subsystem6/2(Out2) -> Subsystem11/1(In1)
  Logical Operator5/1 -> Subsystem3/2(In2)
  Logical Operator7/1 -> Subsystem/2(In2)
  Subsystem11/2(Out2) -> Subsystem9/2(In2)
  Subsystem6/1(Out1) -> Subsystem7/1(In1)
  Subsystem8/1(Out1) -> Subsystem13/1(In1)
  Subsystem13/2(Out2) -> Subsystem12/2(In2)
  Subsystem5/1(Out1) -> Subsystem7/2(In2)
  Logical Operator15/1 -> Subsystem4/1(In1)
  Subsystem3/1(Out1) -> Subsystem4/2(In2)
  Subsystem7/2(Out2) -> Subsystem11/2(In2)
  Subsystem10/1(Out1) -> Subsystem4/3(In3)

== system bit32cpu/ALU/Multiplier/Subsystem2/Subsystem3/Subsystem2 ==
  In1 : Inport
  In2 : Inport  Port=2
  In3 : Inport  Port=3
  In4 : Inport  Port=4
  In5 : Inport  Port=5
  In6 : Inport  Port=6
  In7 : Inport  Port=7
  In8 : Inport  Port=8
  Logical Operator{,1..15} (16 alike) : Logic  AllPortsSameDT=off  OutDataTypeStr=boolean
  Subsystem : Subsystem
  Subsystem1 : Subsystem
  Subsystem10 : Subsystem
  Subsystem11 : Subsystem
  Subsystem12 : Subsystem
  Subsystem13 : Subsystem
  Subsystem14 : Subsystem
  Subsystem2 : Subsystem
  Subsystem3 : Subsystem
  Subsystem4 : Subsystem
  Subsystem5 : Subsystem
  Subsystem6 : Subsystem
  Subsystem7 : Subsystem
  Subsystem8 : Subsystem
  Subsystem9 : Subsystem
  Out1 : Outport
  Out2 : Outport  Port=2
  Out3 : Outport  Port=3
  Out4 : Outport  Port=4
  Out5 : Outport  Port=5
  Out6 : Outport  Port=6
  Out7 : Outport  Port=7
  Out8 : Outport  Port=8
  Out9 : Outport  Port=9
  wires:
  Logical Operator3/1 -> Out9/1
  Subsystem2/1(Out1) -> Out7/1
  Logical Operator4/1 -> Subsystem6/1(In1)
  Subsystem1/2(Out2) -> Subsystem10/1(In1)
  Subsystem9/2(Out2) -> Subsystem14/2(In2)
  Subsystem7/1(Out1) -> Out5/1
  Logical Operator11/1 -> Subsystem1/3(In3)
  Logical Operator10/1 -> Subsystem3/3(In3)
  Subsystem4/1(Out1) -> Out6/1
  In4/1 -> Logical Operator15/2, Logical Operator11/2, Logical Operator7/2, Logical Operator3/2
  Subsystem14/1(Out1) -> Out2/1
  Subsystem14/2(Out2) -> Out1/1
  Logical Operator8/1 -> Subsystem8/1(In1)
  Subsystem3/2(Out2) -> Subsystem5/1(In1)
  In5/1 -> Logical Operator12/1, Logical Operator13/1, Logical Operator14/1, Logical Operator15/1
  In7/1 -> Logical Operator4/1, Logical Operator5/1, Logical Operator6/1, Logical Operator7/1
  Subsystem8/2(Out2) -> Subsystem12/1(In1)
  Subsystem13/1(Out1) -> Out4/1
  Subsystem/1(Out1) -> Out8/1
  Subsystem9/1(Out1) -> Out3/1
  Subsystem11/1(Out1) -> Subsystem8/3(In3)
  Logical Operator2/1 -> Subsystem/1(In1)
  In8/1 -> Logical Operator/1, Logical Operator1/1, Logical Operator2/1, Logical Operator3/1
  Logical Operator6/1 -> Subsystem1/2(In2)
  Subsystem12/1(Out1) -> Subsystem9/3(In3)
  In2/1 -> Logical Operator9/2, Logical Operator13/2, Logical Operator5/2, Logical Operator1/2
  Subsystem5/2(Out2) -> Subsystem13/2(In2)
  Logical Operator12/1 -> Subsystem9/1(In1)
  Subsystem2/2(Out2) -> Subsystem10/2(In2)
  Logical Operator14/1 -> Subsystem6/3(In3)
  In3/1 -> Logical Operator6/2, Logical Operator14/2, Logical Operator10/2, Logical Operator2/2
  Subsystem4/2(Out2) -> Subsystem5/2(In2)
  Subsystem/2(Out2) -> Subsystem2/2(In2)
  In1/1 -> Logical Operator12/2, Logical Operator8/2, Logical Operator4/2, Logical Operator/2
  In6/1 -> Logical Operator8/1, Logical Operator9/1, Logical Operator10/1, Logical Operator11/1
  Logical Operator/1 -> Subsystem3/1(In1)
  Logical Operator9/1 -> Subsystem6/2(In2)
  Subsystem12/2(Out2) -> Subsystem14/1(In1)
  Subsystem10/2(Out2) -> Subsystem7/3(In3)
  Logical Operator13/1 -> Subsystem8/2(In2)
  Logical Operator1/1 -> Subsystem1/1(In1)
  Subsystem1/1(Out1) -> Subsystem2/1(In1)
  Subsystem6/2(Out2) -> Subsystem11/1(In1)
  Logical Operator5/1 -> Subsystem3/2(In2)
  Logical Operator7/1 -> Subsystem/2(In2)
  Subsystem11/2(Out2) -> Subsystem9/2(In2)
  Subsystem6/1(Out1) -> Subsystem7/1(In1)
  Subsystem8/1(Out1) -> Subsystem13/1(In1)
  Subsystem13/2(Out2) -> Subsystem12/2(In2)
  Subsystem5/1(Out1) -> Subsystem7/2(In2)
  Logical Operator15/1 -> Subsystem4/1(In1)
  Subsystem3/1(Out1) -> Subsystem4/2(In2)
  Subsystem7/2(Out2) -> Subsystem11/2(In2)
  Subsystem10/1(Out1) -> Subsystem4/3(In3)

== system bit32cpu/ALU/Multiplier/Subsystem2/Subsystem3/Subsystem3 ==
  In1 : Inport
  In2 : Inport  Port=2
  In3 : Inport  Port=3
  In4 : Inport  Port=4
  In5 : Inport  Port=5
  In6 : Inport  Port=6
  In7 : Inport  Port=7
  In8 : Inport  Port=8
  Logical Operator{,1..15} (16 alike) : Logic  AllPortsSameDT=off  OutDataTypeStr=boolean
  Subsystem : Subsystem
  Subsystem1 : Subsystem
  Subsystem10 : Subsystem
  Subsystem11 : Subsystem
  Subsystem12 : Subsystem
  Subsystem13 : Subsystem
  Subsystem14 : Subsystem
  Subsystem2 : Subsystem
  Subsystem3 : Subsystem
  Subsystem4 : Subsystem
  Subsystem5 : Subsystem
  Subsystem6 : Subsystem
  Subsystem7 : Subsystem
  Subsystem8 : Subsystem
  Subsystem9 : Subsystem
  Out1 : Outport
  Out2 : Outport  Port=2
  Out3 : Outport  Port=3
  Out4 : Outport  Port=4
  Out5 : Outport  Port=5
  Out6 : Outport  Port=6
  Out7 : Outport  Port=7
  Out8 : Outport  Port=8
  Out9 : Outport  Port=9
  wires:
  Logical Operator3/1 -> Out9/1
  Subsystem2/1(Out1) -> Out7/1
  Logical Operator4/1 -> Subsystem6/1(In1)
  Subsystem1/2(Out2) -> Subsystem10/1(In1)
  Subsystem9/2(Out2) -> Subsystem14/2(In2)
  Subsystem7/1(Out1) -> Out5/1
  Logical Operator11/1 -> Subsystem1/3(In3)
  Logical Operator10/1 -> Subsystem3/3(In3)
  Subsystem4/1(Out1) -> Out6/1
  In4/1 -> Logical Operator15/2, Logical Operator11/2, Logical Operator7/2, Logical Operator3/2
  Subsystem14/1(Out1) -> Out2/1
  Subsystem14/2(Out2) -> Out1/1
  Logical Operator8/1 -> Subsystem8/1(In1)
  Subsystem3/2(Out2) -> Subsystem5/1(In1)
  In5/1 -> Logical Operator12/1, Logical Operator13/1, Logical Operator14/1, Logical Operator15/1
  In7/1 -> Logical Operator4/1, Logical Operator5/1, Logical Operator6/1, Logical Operator7/1
  Subsystem8/2(Out2) -> Subsystem12/1(In1)
  Subsystem13/1(Out1) -> Out4/1
  Subsystem/1(Out1) -> Out8/1
  Subsystem9/1(Out1) -> Out3/1
  Subsystem11/1(Out1) -> Subsystem8/3(In3)
  Logical Operator2/1 -> Subsystem/1(In1)
  In8/1 -> Logical Operator/1, Logical Operator1/1, Logical Operator2/1, Logical Operator3/1
  Logical Operator6/1 -> Subsystem1/2(In2)
  Subsystem12/1(Out1) -> Subsystem9/3(In3)
  In2/1 -> Logical Operator9/2, Logical Operator13/2, Logical Operator5/2, Logical Operator1/2
  Subsystem5/2(Out2) -> Subsystem13/2(In2)
  Logical Operator12/1 -> Subsystem9/1(In1)
  Subsystem2/2(Out2) -> Subsystem10/2(In2)
  Logical Operator14/1 -> Subsystem6/3(In3)
  In3/1 -> Logical Operator6/2, Logical Operator14/2, Logical Operator10/2, Logical Operator2/2
  Subsystem4/2(Out2) -> Subsystem5/2(In2)
  Subsystem/2(Out2) -> Subsystem2/2(In2)
  In1/1 -> Logical Operator12/2, Logical Operator8/2, Logical Operator4/2, Logical Operator/2
  In6/1 -> Logical Operator8/1, Logical Operator9/1, Logical Operator10/1, Logical Operator11/1
  Logical Operator/1 -> Subsystem3/1(In1)
  Logical Operator9/1 -> Subsystem6/2(In2)
  Subsystem12/2(Out2) -> Subsystem14/1(In1)
  Subsystem10/2(Out2) -> Subsystem7/3(In3)
  Logical Operator13/1 -> Subsystem8/2(In2)
  Logical Operator1/1 -> Subsystem1/1(In1)
  Subsystem1/1(Out1) -> Subsystem2/1(In1)
  Subsystem6/2(Out2) -> Subsystem11/1(In1)
  Logical Operator5/1 -> Subsystem3/2(In2)
  Logical Operator7/1 -> Subsystem/2(In2)
  Subsystem11/2(Out2) -> Subsystem9/2(In2)
  Subsystem6/1(Out1) -> Subsystem7/1(In1)
  Subsystem8/1(Out1) -> Subsystem13/1(In1)
  Subsystem13/2(Out2) -> Subsystem12/2(In2)
  Subsystem5/1(Out1) -> Subsystem7/2(In2)
  Logical Operator15/1 -> Subsystem4/1(In1)
  Subsystem3/1(Out1) -> Subsystem4/2(In2)
  Subsystem7/2(Out2) -> Subsystem11/2(In2)
  Subsystem10/1(Out1) -> Subsystem4/3(In3)

== system bit32cpu/ALU/Multiplier/Subsystem2/Subsystem3/Subsystem4 ==
  In1 : Inport
  In2 : Inport  Port=2
  In3 : Inport  Port=3
  In4 : Inport  Port=4
  In5 : Inport  Port=5
  In6 : Inport  Port=6
  In7 : Inport  Port=7
  In8 : Inport  Port=8
  In9 : Inport  Port=9
  In10 : Inport  Port=10
  In11 : Inport  Port=11
  In12 : Inport  Port=12
  In13 : Inport  Port=13
  In14 : Inport  Port=14
  In15 : Inport  Port=15
  In16 : Inport  Port=16
  Constant16 : Constant  Value=0
  Subsystem : Subsystem
  Subsystem4 : Subsystem
  Out1 : Outport
  Out2 : Outport  Port=2
  Out3 : Outport  Port=3
  Out4 : Outport  Port=4
  Out5 : Outport  Port=5
  Out6 : Outport  Port=6
  Out7 : Outport  Port=7
  Out8 : Outport  Port=8
  Out9 : Outport  Port=9
  wires:
  Subsystem/3(Out3) -> Out7/1
  Subsystem4/5(Out5) -> Out5/1
  Subsystem4/3(Out3) -> Out3/1
  Subsystem4/1(Out1) -> Out1/1
  Subsystem/2(Out2) -> Out6/1
  Subsystem4/2(Out2) -> Out2/1
  Subsystem/1(Out1) -> Subsystem4/5(In5)
  Subsystem4/4(Out4) -> Out4/1
  Subsystem/5(Out5) -> Out9/1
  Constant16/1 -> Subsystem/5(In5)
  Subsystem/4(Out4) -> Out8/1
  In1/1 -> Subsystem4/1(In1)
  In2/1 -> Subsystem4/2(In2)
  In3/1 -> Subsystem4/3(In3)
  In4/1 -> Subsystem4/4(In4)
  In5/1 -> Subsystem/1(In1)
  In6/1 -> Subsystem/2(In2)
  In7/1 -> Subsystem/3(In3)
  In8/1 -> Subsystem/4(In4)
  In9/1 -> Subsystem4/6(In6)
  In10/1 -> Subsystem4/7(In7)
  In11/1 -> Subsystem4/8(In8)
  In12/1 -> Subsystem4/9(In9)
  In13/1 -> Subsystem/6(In6)
  In14/1 -> Subsystem/7(In7)
  In15/1 -> Subsystem/8(In8)
  In16/1 -> Subsystem/9(In9)

== system bit32cpu/ALU/Multiplier/Subsystem2/Subsystem3/Subsystem5 ==
  In1 : Inport
  In2 : Inport  Port=2
  In3 : Inport  Port=3
  In4 : Inport  Port=4
  In5 : Inport  Port=5
  In6 : Inport  Port=6
  In7 : Inport  Port=7
  In8 : Inport  Port=8
  In9 : Inport  Port=9
  In10 : Inport  Port=10
  In11 : Inport  Port=11
  In12 : Inport  Port=12
  In13 : Inport  Port=13
  In14 : Inport  Port=14
  In15 : Inport  Port=15
  In16 : Inport  Port=16
  Constant16 : Constant  Value=0
  Subsystem : Subsystem
  Subsystem4 : Subsystem
  Out1 : Outport
  Out2 : Outport  Port=2
  Out3 : Outport  Port=3
  Out4 : Outport  Port=4
  Out5 : Outport  Port=5
  Out6 : Outport  Port=6
  Out7 : Outport  Port=7
  Out8 : Outport  Port=8
  Out9 : Outport  Port=9
  wires:
  Subsystem/3(Out3) -> Out7/1
  Subsystem4/5(Out5) -> Out5/1
  Subsystem4/3(Out3) -> Out3/1
  Subsystem4/1(Out1) -> Out1/1
  Subsystem/2(Out2) -> Out6/1
  Subsystem4/2(Out2) -> Out2/1
  Subsystem/1(Out1) -> Subsystem4/5(In5)
  Subsystem4/4(Out4) -> Out4/1
  Subsystem/5(Out5) -> Out9/1
  Constant16/1 -> Subsystem/5(In5)
  Subsystem/4(Out4) -> Out8/1
  In1/1 -> Subsystem4/1(In1)
  In2/1 -> Subsystem4/2(In2)
  In3/1 -> Subsystem4/3(In3)
  In4/1 -> Subsystem4/4(In4)
  In5/1 -> Subsystem/1(In1)
  In6/1 -> Subsystem/2(In2)
  In7/1 -> Subsystem/3(In3)
  In8/1 -> Subsystem/4(In4)
  In9/1 -> Subsystem4/6(In6)
  In10/1 -> Subsystem4/7(In7)
  In11/1 -> Subsystem4/8(In8)
  In12/1 -> Subsystem4/9(In9)
  In13/1 -> Subsystem/6(In6)
  In14/1 -> Subsystem/7(In7)
  In15/1 -> Subsystem/8(In8)
  In16/1 -> Subsystem/9(In9)

== system bit32cpu/ALU/Multiplier/Subsystem2/Subsystem3/Subsystem6 ==
  In1 : Inport
  In2 : Inport  Port=2
  In3 : Inport  Port=3
  In4 : Inport  Port=4
  In5 : Inport  Port=5
  In6 : Inport  Port=6
  In7 : Inport  Port=7
  In8 : Inport  Port=8
  In9 : Inport  Port=9
  In10 : Inport  Port=10
  In11 : Inport  Port=11
  In12 : Inport  Port=12
  In13 : Inport  Port=13
  In14 : Inport  Port=14
  In15 : Inport  Port=15
  In16 : Inport  Port=16
  Constant : Constant  Value=0
  Subsystem : Subsystem
  Subsystem4 : Subsystem
  Out1 : Outport
  Out2 : Outport  Port=2
  Out3 : Outport  Port=3
  Out4 : Outport  Port=4
  Out5 : Outport  Port=5
  Out6 : Outport  Port=6
  Out7 : Outport  Port=7
  Out8 : Outport  Port=8
  Out9 : Outport  Port=9
  wires:
  Subsystem/3(Out3) -> Out7/1
  Subsystem4/5(Out5) -> Out5/1
  Subsystem4/3(Out3) -> Out3/1
  Subsystem4/1(Out1) -> Out1/1
  Subsystem/2(Out2) -> Out6/1
  Subsystem4/2(Out2) -> Out2/1
  Subsystem/1(Out1) -> Subsystem4/5(In5)
  Subsystem4/4(Out4) -> Out4/1
  Subsystem/5(Out5) -> Out9/1
  Constant/1 -> Subsystem/5(In5)
  Subsystem/4(Out4) -> Out8/1
  In1/1 -> Subsystem4/1(In1)
  In2/1 -> Subsystem4/2(In2)
  In3/1 -> Subsystem4/3(In3)
  In4/1 -> Subsystem4/4(In4)
  In5/1 -> Subsystem/1(In1)
  In6/1 -> Subsystem/2(In2)
  In7/1 -> Subsystem/3(In3)
  In8/1 -> Subsystem/4(In4)
  In9/1 -> Subsystem4/6(In6)
  In10/1 -> Subsystem4/7(In7)
  In11/1 -> Subsystem4/8(In8)
  In12/1 -> Subsystem4/9(In9)
  In13/1 -> Subsystem/6(In6)
  In14/1 -> Subsystem/7(In7)
  In15/1 -> Subsystem/8(In8)
  In16/1 -> Subsystem/9(In9)

== system bit32cpu/ALU/Multiplier/Subsystem2/Subsystem4/Subsystem1 ==
  In1 : Inport
  In2 : Inport  Port=2
  In3 : Inport  Port=3
  In4 : Inport  Port=4
  In5 : Inport  Port=5
  In6 : Inport  Port=6
  In7 : Inport  Port=7
  In8 : Inport  Port=8
  Logical Operator{,1..15} (16 alike) : Logic  AllPortsSameDT=off  OutDataTypeStr=boolean
  Subsystem : Subsystem
  Subsystem1 : Subsystem
  Subsystem10 : Subsystem
  Subsystem11 : Subsystem
  Subsystem12 : Subsystem
  Subsystem13 : Subsystem
  Subsystem14 : Subsystem
  Subsystem2 : Subsystem
  Subsystem3 : Subsystem
  Subsystem4 : Subsystem
  Subsystem5 : Subsystem
  Subsystem6 : Subsystem
  Subsystem7 : Subsystem
  Subsystem8 : Subsystem
  Subsystem9 : Subsystem
  Out1 : Outport
  Out2 : Outport  Port=2
  Out3 : Outport  Port=3
  Out4 : Outport  Port=4
  Out5 : Outport  Port=5
  Out6 : Outport  Port=6
  Out7 : Outport  Port=7
  Out8 : Outport  Port=8
  Out9 : Outport  Port=9
  wires:
  Logical Operator3/1 -> Out9/1
  Subsystem2/1(Out1) -> Out7/1
  Logical Operator4/1 -> Subsystem6/1(In1)
  Subsystem1/2(Out2) -> Subsystem10/1(In1)
  Subsystem9/2(Out2) -> Subsystem14/2(In2)
  Subsystem7/1(Out1) -> Out5/1
  Logical Operator11/1 -> Subsystem1/3(In3)
  Logical Operator10/1 -> Subsystem3/3(In3)
  Subsystem4/1(Out1) -> Out6/1
  In4/1 -> Logical Operator15/2, Logical Operator11/2, Logical Operator7/2, Logical Operator3/2
  Subsystem14/1(Out1) -> Out2/1
  Subsystem14/2(Out2) -> Out1/1
  Logical Operator8/1 -> Subsystem8/1(In1)
  Subsystem3/2(Out2) -> Subsystem5/1(In1)
  In5/1 -> Logical Operator12/1, Logical Operator13/1, Logical Operator14/1, Logical Operator15/1
  In7/1 -> Logical Operator4/1, Logical Operator5/1, Logical Operator6/1, Logical Operator7/1
  Subsystem8/2(Out2) -> Subsystem12/1(In1)
  Subsystem13/1(Out1) -> Out4/1
  Subsystem/1(Out1) -> Out8/1
  Subsystem9/1(Out1) -> Out3/1
  Subsystem11/1(Out1) -> Subsystem8/3(In3)
  Logical Operator2/1 -> Subsystem/1(In1)
  In8/1 -> Logical Operator/1, Logical Operator1/1, Logical Operator2/1, Logical Operator3/1
  Logical Operator6/1 -> Subsystem1/2(In2)
  Subsystem12/1(Out1) -> Subsystem9/3(In3)
  In2/1 -> Logical Operator9/2, Logical Operator13/2, Logical Operator5/2, Logical Operator1/2
  Subsystem5/2(Out2) -> Subsystem13/2(In2)
  Logical Operator12/1 -> Subsystem9/1(In1)
  Subsystem2/2(Out2) -> Subsystem10/2(In2)
  Logical Operator14/1 -> Subsystem6/3(In3)
  In3/1 -> Logical Operator6/2, Logical Operator14/2, Logical Operator10/2, Logical Operator2/2
  Subsystem4/2(Out2) -> Subsystem5/2(In2)
  Subsystem/2(Out2) -> Subsystem2/2(In2)
  In1/1 -> Logical Operator12/2, Logical Operator8/2, Logical Operator4/2, Logical Operator/2
  In6/1 -> Logical Operator8/1, Logical Operator9/1, Logical Operator10/1, Logical Operator11/1
  Logical Operator/1 -> Subsystem3/1(In1)
  Logical Operator9/1 -> Subsystem6/2(In2)
  Subsystem12/2(Out2) -> Subsystem14/1(In1)
  Subsystem10/2(Out2) -> Subsystem7/3(In3)
  Logical Operator13/1 -> Subsystem8/2(In2)
  Logical Operator1/1 -> Subsystem1/1(In1)
  Subsystem1/1(Out1) -> Subsystem2/1(In1)
  Subsystem6/2(Out2) -> Subsystem11/1(In1)
  Logical Operator5/1 -> Subsystem3/2(In2)
  Logical Operator7/1 -> Subsystem/2(In2)
  Subsystem11/2(Out2) -> Subsystem9/2(In2)
  Subsystem6/1(Out1) -> Subsystem7/1(In1)
  Subsystem8/1(Out1) -> Subsystem13/1(In1)
  Subsystem13/2(Out2) -> Subsystem12/2(In2)
  Subsystem5/1(Out1) -> Subsystem7/2(In2)
  Logical Operator15/1 -> Subsystem4/1(In1)
  Subsystem3/1(Out1) -> Subsystem4/2(In2)
  Subsystem7/2(Out2) -> Subsystem11/2(In2)
  Subsystem10/1(Out1) -> Subsystem4/3(In3)
